simulink model "simulink_testfile_pt2"  (R2017a)
settings: Solver=ode45  StartTime=0.0  StopTime=10.0  RelTol=1e-3  EnableMultiTasking=on
values from neighbouring files (symbols this model uses):
  T = 0.5    [set_parameter_pt2.m]
  V = 2    [set_parameter_pt2.m]
  xi = 0.2    [set_parameter_pt2.m]
settings Model: Creator=rolex  LastModifiedBy=maam
settings DataIOCC: LimitDataPoints=on  SaveFormat=Array
settings OptimizationCC: ExpressionDepthLimit=2147483647  LifeSpan=inf
settings DebuggingCC: UnderspecifiedInitializationDetection=Classic  MergeDetectMultiDrivingBlocksExec=none  SolverPrmCheckMsg=warning  StateNameClashWarn=warning  SFUnexpectedBacktrackingDiag=warning  SFNoUnconditionalDefaultTransitionDiag=warning  SFExecutionAtInitializationDiag=none
settings HardwareCC: ProdBitPerPointer=32  ProdBitPerSizeT=32  ProdBitPerPtrDiffT=32  ProdLargestAtomicFloat=None  ProdIntDivRoundTo=Undefined  ProdEndianess=Unspecified  ProdWordSize=32  ProdHWDeviceType=32-bit Generic
settings ModelReferenceCC: PropagateSignalLabelsOutOfModel=off
settings GRTTargetCC: TargetLangStandard=C89/C90 (ANSI)  GeneratePreprocessorConditionals=Disable all
settings ConfigComp: CovMetricSettings=dw  CovHtmlReporting=on  CovSaveCumulativeToWorkspaceVar=on  CovSaveSingleToWorkspaceVar=on  CovExternalEMLEnable=off

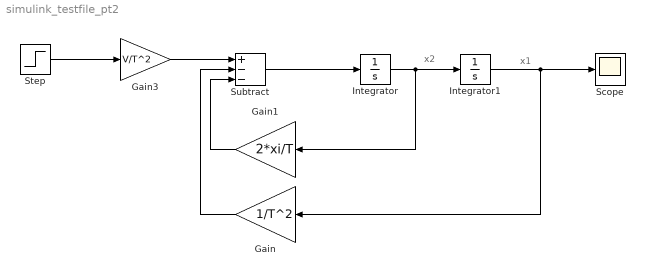
== system simulink_testfile_pt2 ==
  note: x2
  note: x1
  Gain : Gain  Gain=1/T^2
  Gain1 : Gain  Gain=2*xi/T
  Gain3 : Gain  Gain=V/T^2
  Integrator : Integrator
  Integrator1 : Integrator
  Scope : Scope
  Step : Step  SampleTime=0
  Subtract : Sum  Inputs=+--
  wires:
  Subtract/1 -> Integrator/1
  Integrator/1 -> Integrator1/1, Gain1/1
  Gain1/1 -> Subtract/3
  Gain/1 -> Subtract/2
  Integrator1/1 -> Scope/1, Gain/1
  Gain3/1 -> Subtract/1
  Step/1 -> Gain3/1
